simulink model "CAN_Model_v2"  (R2018b)
settings: Solver=VariableStepAuto  StartTime=0.0  StopTime=20  RelTol=1e-3
libraries: simulink_extras x1
settings Model: Creator=Emiliano  LastModifiedBy=Emiliano

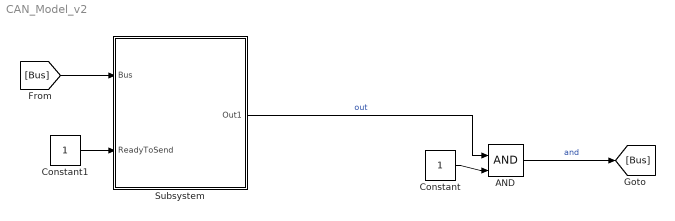
== system CAN_Model_v2 ==
  AND : Logic  IconShape=distinctive  AllPortsSameDT=off  OutDataTypeStr=boolean
  Constant : Constant  SampleTime=0.2
  Constant1 : Constant
  Subsystem : Subsystem
  wires:
  Subsystem/1(Out1) -> AND/1  "out"
  Constant/1 -> AND/2
  AND/1 -> [Bus]  "and"
  [Bus] -> Subsystem/1(Bus)
  Constant1/1 -> Subsystem/2("ReadyToSend ")

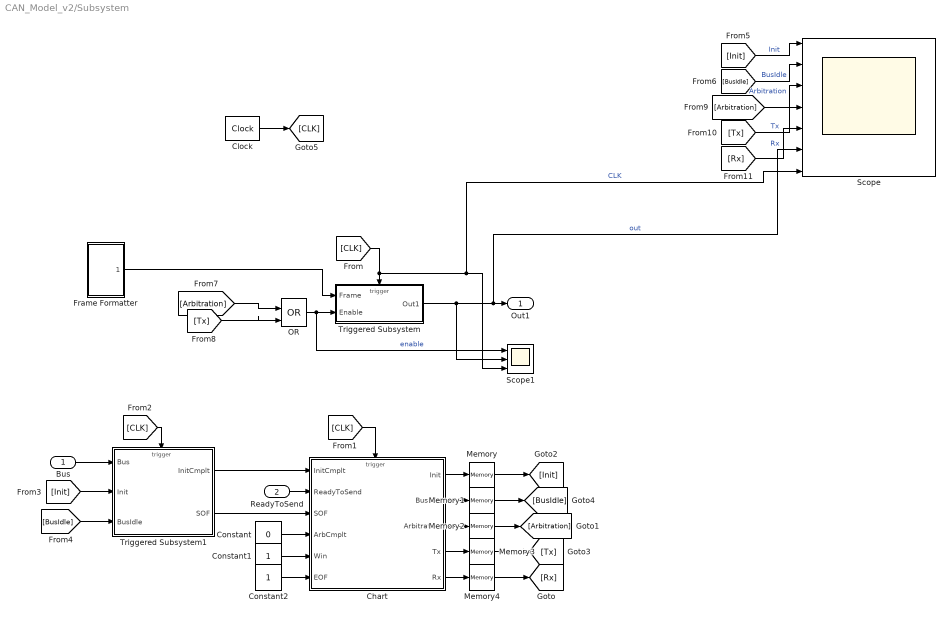
== system CAN_Model_v2/Subsystem ==
  Bus : Inport
  "ReadyToSend " : Inport  Port=2
  Chart : Stateflow chart  TreatAsAtomicUnit=on
  Clock : simulink_extras/Flip Flops/Clock  period=0.2
  Constant : Constant  Value=0
  Constant1 : Constant
  Constant2 : Constant
  Frame Formatter : Subsystem
  Memory{,1..4} (5 alike) : Memory
  OR : Logic  Operator=OR  IconShape=distinctive  AllPortsSameDT=off  OutDataTypeStr=boolean
  Scope : Scope  NumInputPorts=7
  Scope1 : Scope  NumInputPorts=3
  Triggered Subsystem : Subsystem  TreatAsAtomicUnit=on
  Triggered Subsystem1 : Subsystem  TreatAsAtomicUnit=on
  Out1 : Outport
  wires:
  [CLK] -> Chart/Trigger
  [Arbitration] -> OR/1
  [Tx] -> OR/2
  Frame Formatter/1(Frame) -> Triggered Subsystem/1("Frame ")
  OR/1 -> Scope1/1, Triggered Subsystem/2(Enable)  "enable"
  Chart/5(" Rx") -> Memory4/1
  Chart/3(" Arbitration") -> Memory2/1
  Chart/1(" Init") -> Memory/1
  Chart/4(" Tx") -> Memory3/1
  Chart/2(" BusIdle") -> Memory1/1
  Clock/1 -> [CLK]
  [CLK] -> Scope/7, Scope1/3, Triggered Subsystem/Trigger  "CLK"
  [CLK] -> Triggered Subsystem1/Trigger
  Triggered Subsystem1/1(InitCmplt) -> Chart/1(InitCmplt)
  Bus/1 -> Triggered Subsystem1/1(Bus)
  [Init] -> Triggered Subsystem1/2(Init)
  "ReadyToSend "/1 -> Chart/2(ReadyToSend)
  [BusIdle] -> Triggered Subsystem1/3(BusIdle)
  Triggered Subsystem1/2(SOF) -> Chart/3(SOF)
  Constant2/1 -> Chart/6(EOF)
  Constant1/1 -> Chart/5(Win)
  Constant/1 -> Chart/4(ArbCmplt)
  [Init] -> Scope/1  "Init"
  [BusIdle] -> Scope/2  "BusIdle"
  [Arbitration] -> Scope/3  "Arbitration"
  [Tx] -> Scope/4  "Tx"
  [Rx] -> Scope/5  "Rx"
  Memory/1 -> [Init]
  Memory1/1 -> [BusIdle]
  Memory2/1 -> [Arbitration]
  Memory3/1 -> [Tx]
  Memory4/1 -> [Rx]
  Triggered Subsystem/1(Out1) -> Scope1/2, Scope/6, Out1/1  "out"

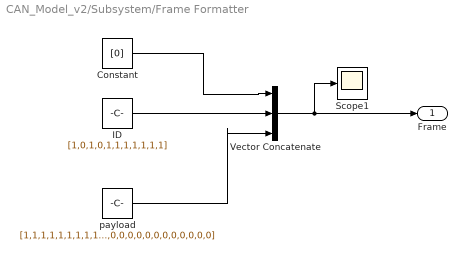
== system CAN_Model_v2/Subsystem/Frame Formatter ==
  Constant : Constant  Value=[0]
  ID : Constant  Value=[1,0,1,0,1,1,1,1,1,1,1]
  Scope1 : Scope
  Vector Concatenate : Concatenate  NumInputs=3
  "payload " : Constant  Value=[1,1,1,1,1,1,1,1,1,1,1,1,1,1,1,1,1,1,1,1,1,1,1,1,1,0,0,0,0,0,0,0,0,0,0,0,0,0,0,0,0,0,0,0,0,0,0,0,0,0]
  Frame : Outport
  wires:
  ID/1 -> Vector Concatenate/2
  Constant/1 -> Vector Concatenate/1
  "payload "/1 -> Vector Concatenate/3
  Vector Concatenate/1 -> Frame/1, Scope1/1

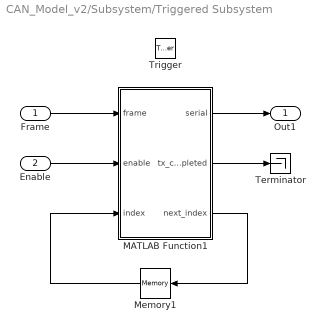
== system CAN_Model_v2/Subsystem/Triggered Subsystem ==
  "Frame " : Inport
  Enable : Inport  Port=2
  Trigger : TriggerPort  VariantControl=Variant
  MATLAB Function1 : MATLAB Function  TreatAsAtomicUnit=on
  Memory1 : Memory  InitialCondition=1  InheritSampleTime=on
  Terminator : Terminator
  Out1 : Outport
  wires:
  "Frame "/1 -> MATLAB Function1/1(frame)
  Memory1/1 -> MATLAB Function1/3(index)
  MATLAB Function1/1(serial) -> Out1/1
  MATLAB Function1/3(next_index) -> Memory1/1
  MATLAB Function1/2(tx_completed) -> Terminator/1
  Enable/1 -> MATLAB Function1/2(enable)

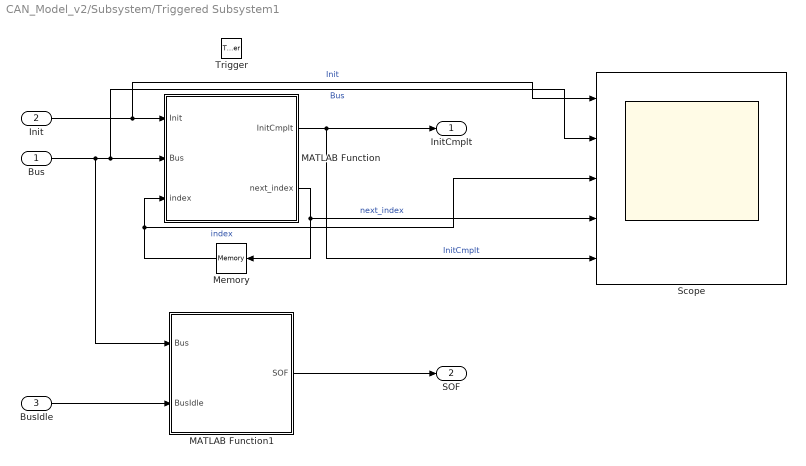
== system CAN_Model_v2/Subsystem/Triggered Subsystem1 ==
  Bus : Inport
  Init : Inport  Port=2
  BusIdle : Inport  Port=3
  Trigger : TriggerPort  VariantControl=Variant
  MATLAB Function : MATLAB Function  TreatAsAtomicUnit=on
  MATLAB Function1 : MATLAB Function  TreatAsAtomicUnit=on
  Memory : Memory  InheritSampleTime=on
  Scope : Scope  NumInputPorts=5
  InitCmplt : Outport
  SOF : Outport  Port=2
  wires:
  MATLAB Function/2(next_index) -> Scope/4, Memory/1  "next_index"
  Memory/1 -> Scope/3, MATLAB Function/3(index)  "index"
  Bus/1 -> MATLAB Function1/1(Bus), Scope/2, MATLAB Function/2(Bus)  "Bus"
  MATLAB Function/1(InitCmplt) -> InitCmplt/1, Scope/5  "InitCmplt"
  MATLAB Function1/1(SOF) -> SOF/1
  Init/1 -> Scope/1, MATLAB Function/1(Init)  "Init"
  BusIdle/1 -> MATLAB Function1/2(BusIdle)

== matlab function CAN_Model_v2/Subsystem/Triggered Subsystem1/MATLAB Function ==
  data: Init input; InitCmplt output; Bus input; index input; next_index output
function [InitCmplt, next_index] = BusIdleSensing(Init, Bus, index)

InitCmplt = 0;

if Init == 1
    if Bus == 1
        if index < 10 %Number of one to wait for EOF (after 11 ones)
            next_index = index + 1;
        else
            next_index = 0;
            InitCmplt = 1;
        end
    else
        next_index = 0;
    end
else
   next_index = 0;
end

end

== matlab function CAN_Model_v2/Subsystem/Triggered Subsystem/MATLAB Function1 ==
  data: frame input; enable input; serial output; tx_completed output; index input; next_index output
function [serial,  tx_completed ,next_index]  = fcn(frame, enable, index)

if enable == 1
    frame_size = length(frame);
    if index > frame_size
        serial = 1;
        tx_completed = 1;
        next_index = 1;
    else
        serial = frame(index);
        next_index = index + 1;
        tx_completed = 0;
    end
else
    tx_completed = 0;
    serial = 1;
    next_index = 1;
end

end

== stateflow chart CAN_Model_v2/Subsystem/Chart ==
  settings: sampleTime=0.2  executeAtInitialization=1
  state Init
  state Rx
  state BusIdle
  state Arbitration
  state Tx
  Init -> Init [order 2] : [InitCmplt == 0]
  (default) -> Init
  Init -> BusIdle [order 1] : [InitCmplt == 1]
  Rx -> Rx [order 2] : [EOF == 0]
  BusIdle -> Rx [order 2] : [ReadyToSend == 0 && SOF == 1]
  Rx -> BusIdle [order 1] : [EOF == 1]
  BusIdle -> BusIdle [order 3] : [ReadyToSend == 0 && SOF == 0]
  Arbitration -> Rx [order 1] : [ArbCmplt ==1 && Win == 0]
  Tx -> BusIdle [order 2] : [EOF == 1]
  BusIdle -> Arbitration [order 1] : [ReadyToSend > 0]
  Arbitration -> Tx [order 2] : [ArbCmplt ==1 && Win == 1]
  Arbitration -> Arbitration [order 3] : [ArbCmplt == 0]
  Tx -> Tx [order 1] : [EOF == 0]
  data: Init output boolean; BusIdle output boolean; Arbitration output boolean; Tx output boolean; Rx output boolean; InitCmplt input; ReadyToSend input; SOF input; ArbCmplt input; Win input; EOF input
  events: Start input FALLING_EDGE_EVENT

== matlab function CAN_Model_v2/Subsystem/Triggered Subsystem1/MATLAB Function1 ==
  data: Bus input; SOF output; BusIdle input
function SOF = SOF_Detection(Bus, BusIdle)

if BusIdle == 1 %Checks the current state of the FSM
    if Bus == 0
        SOF = 1; %SOF Detected, the flag goes to One!
    else
        SOF = 0;    
    end
else
    SOF = 0;
end

end
